simulink model "ReplayFlight_ALL_PARMS_v6"  (Simulink 7.5)
settings: Solver=FixedStepDiscrete  StartTime=0.0  StopTime=d_data(end,1)  FixedStep=apSampleTime  RelTol=1e-3
InitFcn:
  | replayFlight
values from neighbouring files (symbols this model uses):
  apSampleTime = 0.01    [demoz2SlugsV5.m]
  D = y    [BarOrthog.m]
  QUAT_0 = DCM2Quat( R0 )    [demoz2SlugsV5.m]
  R0 = single(Euler2DCMdeg( PHI_IC, THETA_IC, PSI_IC ))    [demoz2SlugsV5.m]
  SampleT = 0.02    [demoz2SlugsV5.m]
undefined symbols (not defined in the file or in its folder): aAxis_IC, accBiasRateLimit, accelXCutTemp, aPhi_IC, axTGain1, axTGain2, axTMean1, axTMean2, barAdjust, baroCutoff, baroCutTemp, baroOffset, baroScale, barTGain1, barTGain2, barTMean1, barTMean2, baseHeight, baseTemp, cubeAccelGain, cubeGyroGain, DiscIntNeverNeededParam, ePhi_IC, gaind, GS_location, gyroBiasRateLimit, Init_onlyOnce, Init_Reset, ISA_rho0, lapseRate, lowRateSensorCutoff, magMeanTemp, magOffset, magScale, magTempK, mainSensorCutoff, maxDynPressure, param_acc, param_mag, pitAdjust, pitCutTemp, pitotOffset, pitotScale, pitTGain1, pitTGain2, pitTMean1, pitTMean2, polesd, powerOffset, powerScale, pressureSensorCutoff, Psi_IC, T, tempOffset, tempScale, Theta_IC, Vb_0, vzCutoff, xCutoff, yCutoff ... (+2)
libraries: simulink x38, aerolibconvert2 x8, SLUGS_Library x6, dspmtrx3 x5, aerolibutil x4, dsPICdrivers x1
(part 4 of 5)

== system ReplayFlight_ALL_PARMS_v6/Position and Attitude Filter/Attitude Complimentary Filter COG/DoParmTests/DCM Tests/Create_OmegaBar ==
  w_curr : Inport
  w_prev : Inport  Port=2
  w_prev2 : Inport  Port=3
  2xapSampleTime : Constant  Value=2*apSampleTime  OutDataTypeMode=single  OutDataType=fixdt(1, 16)  OutScaling=2^0  OutDataTypeStr=single
  Const_2 : Constant  Value=2  OutDataTypeMode=single  OutDataType=fixdt(1, 16)  OutScaling=2^0  OutDataTypeStr=single
  Constant_1_2 : Constant  Value=1/2  OutDataTypeMode=single  OutDataType=fixdt(1, 16)  OutScaling=2^0  OutDataTypeStr=single
  Constant_1_6 : Constant  Value=1/6  OutDataTypeMode=single  OutDataType=fixdt(1, 16)  OutScaling=2^0  OutDataTypeStr=single
  Oddot : Product  Inputs=*/  OutDataType=fixdt(1, 16)  OutScaling=2^-10
  Odot : Product  Inputs=*/  OutDataType=fixdt(1, 16)  OutScaling=2^-10
  Product : Product  OutDataType=fixdt(1, 16)  OutScaling=2^0  RndMeth=Zero
  Product1 : Product  Inputs=3  OutDataType=fixdt(1, 16)  OutScaling=2^0  RndMeth=Zero
  Product2 : Product  Inputs=3  OutDataType=fixdt(1, 16)  OutScaling=2^0  RndMeth=Zero
  Product3 : Product  OutDataTypeMode=single  OutDataType=fixdt(1, 16)  OutScaling=2^0  OutDataTypeStr=single  SampleTime=apSampleTime  RndMeth=Zero
  SampleTime_sqrd : Constant  Value=apSampleTime^2  OutDataTypeMode=single  OutDataType=fixdt(1, 16)  OutScaling=2^0  OutDataTypeStr=single
  Subtract : Sum  Inputs=+-  OutDataType=fixdt(1, 16)  OutScaling=2^-10
  Subtract1 : Sum  Inputs=+-+  OutDataType=fixdt(1, 16)  OutScaling=2^-10
  Subtract2 : Sum  Inputs=+++  OutDataTypeMode=single  OutDataType=fixdt(1, 16)  OutScaling=2^-10  OutDataTypeStr=single
  apSampleTime : Constant  Value=apSampleTime  OutDataTypeMode=single  OutDataType=fixdt(1, 16)  OutScaling=2^0  OutDataTypeStr=single
  OmegaBar : Outport
  wires:
  Product2/1 -> Subtract2/3
  Oddot/1 -> Product2/2
  Product3/1 -> Product2/1
  Constant_1_6/1 -> Product2/3
  Product1/1 -> Subtract2/2
  Odot/1 -> Product1/3
  apSampleTime/1 -> Product3/2, Product3/1, Product1/2
  Constant_1_2/1 -> Product1/1
  Subtract2/1 -> OmegaBar/1
  Product/1 -> Subtract1/2
  Const_2/1 -> Product/2
  Subtract1/1 -> Oddot/1
  SampleTime_sqrd/1 -> Oddot/2
  2xapSampleTime/1 -> Odot/2
  Subtract/1 -> Odot/1
  w_prev2/1 -> Subtract1/3, Subtract/2
  w_curr/1 -> Subtract1/1, Subtract/1
  w_prev/1 -> Subtract2/1, Product/1

== system ReplayFlight_ALL_PARMS_v6/Position and Attitude Filter/Attitude Complimentary Filter COG/DoParmTests/DCM Tests/Murray_Mexp ==
  w_in : Inport  OutDataType=fixdt(1, 16)  OutScaling=2^0
  R_prev : Inport  Port=2  OutDataType=fixdt(1, 16)  OutScaling=2^0
  Add : Sum  Inputs=+++  OutDataTypeMode=single  OutDataType=fixdt(1, 16)  OutScaling=2^-10  OutDataTypeStr=single  SampleTime=apSampleTime
  Cosine_X : Trigonometry  Operator=cos
  Divide : Product  Inputs=*/  OutDataType=fixdt(1, 16)  OutScaling=2^-10
  Divide1 : Product  Inputs=*/  OutDataType=fixdt(1, 16)  OutScaling=2^-10
  Embedded MATLAB Function : Stateflow chart  TreatAsAtomicUnit=on
  Identity Matrix : dspmtrx3/Identity Matrix  Inherit=off  N=3  Ts=apSampleTime  dataType=single  isSigned=on  wordLen=16  udDataType=sfix(16)  fracBitsMode=Best precision  numFracBits=15
  Identity Matrix1 : dspmtrx3/Identity Matrix  Inherit=off  N=3  Ts=apSampleTime  dataType=single  isSigned=on  wordLen=16  udDataType=sfix(16)  fracBitsMode=Best precision  numFracBits=15
  Matrix Multiply1 : Product  Multiplication=Matrix(*)  OutDataType=sfix(16)  OutScaling=2^0
  Matrix Multiply2 : Product  Multiplication=Matrix(*)  OutDataType=sfix(16)  OutScaling=2^0
  Product{,1..3} (4 alike) : Product  OutDataType=fixdt(1, 16)  OutScaling=2^0  RndMeth=Zero
  Rexp : Switch  Criteria=u2 ~= 0  OutDataType=fixdt(1, 16)  OutScaling=2^0
  Sine_X : Trigonometry
  Skew symmetric matrix : Subsystem
  Subtract : Sum  Inputs=+-  OutDataType=fixdt(1, 16)  OutScaling=2^-10
  apSampleTime : Constant  Value=apSampleTime  OutDataTypeMode=single  OutDataType=fixdt(1, 16)  OutScaling=2^0  OutDataTypeStr=single
  apSampleTime1 : Constant  OutDataTypeMode=single  OutDataType=fixdt(1, 16)  OutScaling=2^0  OutDataTypeStr=single
  DCM_out : Outport  OutDataType=fixdt(1, 16)  OutScaling=2^0
  wires:
  Rexp/1 -> Matrix Multiply1/2
  Identity Matrix1/1 -> Rexp/3
  Add/1 -> Rexp/1
  Matrix Multiply1/1 -> DCM_out/1
  R_prev/1 -> Matrix Multiply1/1
  Product3/1 -> Add/2
  Divide/1 -> Product3/2
  Sine_X/1 -> Divide/1
  Product2/1 -> Add/3
  Matrix Multiply2/1 -> Product2/1
  Divide1/1 -> Product2/2
  Product1/1 -> Divide1/2
  Subtract/1 -> Divide1/1
  Cosine_X/1 -> Subtract/2
  apSampleTime1/1 -> Subtract/1
  Skew symmetric matrix/1(omega_x) -> Product3/1, Matrix Multiply2/2, Matrix Multiply2/1
  Product/1 -> Sine_X/1, Cosine_X/1
  apSampleTime/1 -> Product/2
  Embedded MATLAB Function/1(y) -> Rexp/2, Divide/2, Product1/1, Product1/2, Product/1
  Identity Matrix/1 -> Add/1
  w_in/1 -> Embedded MATLAB Function/1(u), Skew symmetric matrix/1(omega_in)

== system ReplayFlight_ALL_PARMS_v6/Position and Attitude Filter/Attitude Complimentary Filter COG/DoParmTests/DCM Tests/Skew symmetric matrix ==
  omega_in : Inport  PortDimensions=3  SampleTime=SampleT  OutDataType=fixdt(1, 16)  OutScaling=2^0
  Constant : Constant  Value=0  OutDataTypeMode=single  OutDataType=fixdt(1, 16)  OutScaling=2^0  OutDataTypeStr=single
  Constant1 : Constant  Value=0  OutDataTypeMode=single  OutDataType=fixdt(1, 16)  OutScaling=2^0  OutDataTypeStr=single
  Constant2 : Constant  Value=0  OutDataTypeMode=single  OutDataType=fixdt(1, 16)  OutScaling=2^0  OutDataTypeStr=single
  Demux : Demux  Outputs=3
  Gain : Gain  Gain=-1  ParameterDataType=fixdt(1, 16)  ParameterScaling=2^0  OutDataType=fixdt(1, 16)  OutScaling=2^0
  Gain1 : Gain  Gain=-1  ParameterDataType=fixdt(1, 16)  ParameterScaling=2^0  OutDataType=fixdt(1, 16)  OutScaling=2^0
  Gain2 : Gain  Gain=-1  ParameterDataType=fixdt(1, 16)  ParameterScaling=2^0  OutDataType=fixdt(1, 16)  OutScaling=2^0
  Mux{,1..3} (4 alike) : Mux  Inputs=3
  Reshape : Reshape  OutputDimensionality=Customize  OutputDimensions=[3,3]
  omega_x : Outport  PortDimensions=[3,3]  SampleTime=SampleT  OutDataType=fixdt(1, 16)  OutScaling=2^0
  wires:
  Gain2/1 -> Mux2/2
  Gain1/1 -> Mux1/1
  Gain/1 -> Mux/3
  Mux3/1 -> Reshape/1
  Mux2/1 -> Mux3/3
  Mux1/1 -> Mux3/2
  Mux/1 -> Mux3/1
  Constant2/1 -> Mux2/3
  Demux/1 -> Gain2/1, Mux1/3
  Constant1/1 -> Mux1/2
  Demux/2 -> Mux2/1, Gain/1
  Demux/3 -> Gain1/1, Mux/2
  Constant/1 -> Mux/1
  Reshape/1 -> omega_x/1
  omega_in/1 -> Demux/1

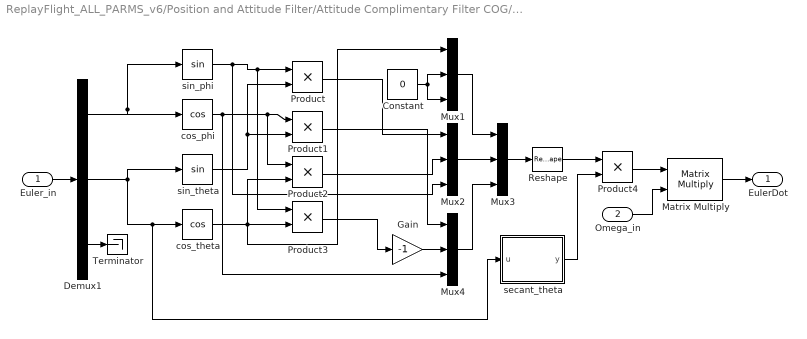
== system ReplayFlight_ALL_PARMS_v6/Position and Attitude Filter/Attitude Complimentary Filter COG/DoParmTests/Euler_Test/CreateEulerDot ==
  Euler_in : Inport  PortDimensions=3  SampleTime=SampleT  DataType=single  OutDataType=fixdt(1, 16)  OutScaling=2^0  OutDataTypeStr=single
  Omega_in : Inport  Port=2  PortDimensions=[3,1]  SampleTime=SampleT  DataType=single  OutDataType=fixdt(1, 16)  OutScaling=2^0  OutDataTypeStr=single
  Constant : Constant  Value=0  OutDataTypeMode=single  OutDataType=fixdt(1, 16)  OutScaling=2^0  OutDataTypeStr=single  SampleTime=SampleT
  Demux1 : Demux  Outputs=3
  Gain : Gain  Gain=-1  ParameterDataType=fixdt(1, 16)  ParameterScaling=2^0  OutDataTypeMode=single  OutDataType=fixdt(1, 16)  OutScaling=2^0  OutDataTypeStr=single  SampleTime=SampleT
  Matrix Multiply : Product  Multiplication=Matrix(*)  OutDataTypeMode=single  OutDataType=sfix(16)  OutScaling=2^0  OutDataTypeStr=single
  Mux{1..4} (4 alike) : Mux  Inputs=3
  Product{,1..3} (4 alike) : Product  OutDataTypeMode=single  OutDataType=fixdt(1, 16)  OutScaling=2^0  OutDataTypeStr=single  RndMeth=Zero
  Product4 : Product  OutDataTypeMode=single  OutDataType=fixdt(1, 16)  OutScaling=2^0  OutDataTypeStr=single  SampleTime=SampleT  RndMeth=Zero
  Reshape : Reshape  OutputDimensionality=Customize  OutputDimensions=[3,3]
  Terminator : Terminator
  cos_phi : Trigonometry  Operator=cos  SampleTime=SampleT
  cos_theta : Trigonometry  Operator=cos  SampleTime=SampleT
  secant_theta : Stateflow chart  TreatAsAtomicUnit=on
  sin_phi : Trigonometry  SampleTime=SampleT
  sin_theta : Trigonometry  SampleTime=SampleT
  EulerDot : Outport  DataType=single  OutDataType=fixdt(1, 16)  OutScaling=2^0  OutDataTypeStr=single
  wires:
  Product4/1 -> Matrix Multiply/1
  Reshape/1 -> Product4/1
  secant_theta/1(y) -> Product4/2
  Product3/1 -> Gain/1
  Gain/1 -> Mux4/2
  Product1/1 -> Mux4/1
  Product2/1 -> Mux2/2
  Product/1 -> Mux2/1
  Constant/1 -> Mux1/3, Mux1/2
  Mux4/1 -> Mux3/3
  Mux2/1 -> Mux3/2
  Mux1/1 -> Mux3/1
  Mux3/1 -> Reshape/1
  Omega_in/1 -> Matrix Multiply/2
  Matrix Multiply/1 -> EulerDot/1
  cos_theta/1 -> Mux1/1, Product3/2, Product2/2
  cos_phi/1 -> Mux4/3, Product2/1, Product1/1
  sin_theta/1 -> Product1/2, Product/2
  sin_phi/1 -> Mux2/3, Product3/1, Product/1
  Demux1/2 -> secant_theta/1(u), cos_theta/1, sin_theta/1
  Demux1/1 -> cos_phi/1, sin_phi/1
  Demux1/3 -> Terminator/1
  Euler_in/1 -> Demux1/1

== system ReplayFlight_ALL_PARMS_v6/Position and Attitude Filter/Attitude Complimentary Filter COG/DoParmTests/Euler_Test/Create_OmegaAverage ==
  In1 : Inport
  In2 : Inport  Port=2
  Add : Sum  OutDataType=fixdt(1, 16)  OutScaling=2^-10
  Constant : Constant  Value=2  OutDataTypeMode=single  OutDataType=fixdt(1, 16)  OutScaling=2^0  OutDataTypeStr=single
  Divide : Product  Inputs=*/  OutDataType=fixdt(1, 16)  OutScaling=2^-10
  Out1 : Outport
  wires:
  Constant/1 -> Divide/2
  Add/1 -> Divide/1
  In1/1 -> Add/1
  In2/1 -> Add/2
  Divide/1 -> Out1/1

== system ReplayFlight_ALL_PARMS_v6/Position and Attitude Filter/Attitude Complimentary Filter COG/DoParmTests/Euler_Test/Euler2DCM ==
  Euler_in : Inport  PortDimensions=3
  Create 3x3 Matrix : aerolibutil/Create 3x3 Matrix  SystemSampleTime=-1
  Fcn : Fcn  Expr=u(6)*u(5)  SampleTime=apSampleTime
  Fcn1 : Fcn  Expr=u(6)*u(2)*u(1)-u(3)*u(4)  SampleTime=apSampleTime
  Fcn2 : Fcn  Expr=u(6)*u(2)*u(4)+u(3)*u(1)  SampleTime=apSampleTime
  Fcn3 : Fcn  Expr=u(3)*u(5)  SampleTime=apSampleTime
  Fcn4 : Fcn  Expr=u(3)*u(2)*u(1)+u(6)*u(4)  SampleTime=apSampleTime
  Fcn5 : Fcn  Expr=u(3)*u(2)*u(4)-u(6)*u(1)  SampleTime=apSampleTime
  Fcn6 : Fcn  Expr=-u(2)  SampleTime=apSampleTime
  Fcn7 : Fcn  Expr=u(5)*u(1)  SampleTime=apSampleTime
  Fcn8 : Fcn  Expr=u(5)*u(4)  SampleTime=apSampleTime
  Mux1 : Mux  Inputs=2
  sincos : Trigonometry  Operator=sincos
  eDCM_out : Outport  PortDimensions=[3,3]
  wires:
  Euler_in/1 -> sincos/1
  sincos/1 -> Mux1/1
  sincos/2 -> Mux1/2
  Create 3x3 Matrix/1 -> eDCM_out/1
  Mux1/1 -> Fcn/1, Fcn1/1, Fcn2/1, Fcn3/1, Fcn4/1, Fcn5/1, Fcn8/1, Fcn7/1, Fcn6/1
  Fcn/1 -> Create 3x3 Matrix/1
  Fcn1/1 -> Create 3x3 Matrix/2
  Fcn2/1 -> Create 3x3 Matrix/3
  Fcn3/1 -> Create 3x3 Matrix/4
  Fcn4/1 -> Create 3x3 Matrix/5
  Fcn5/1 -> Create 3x3 Matrix/6
  Fcn6/1 -> Create 3x3 Matrix/7
  Fcn7/1 -> Create 3x3 Matrix/8
  Fcn8/1 -> Create 3x3 Matrix/9

== system ReplayFlight_ALL_PARMS_v6/Position and Attitude Filter/Attitude Complimentary Filter COG/DoParmTests/Quat_Test/Create_OmegaAverage ==
  In1 : Inport
  In2 : Inport  Port=2
  Add : Sum  OutDataType=fixdt(1, 16)  OutScaling=2^-10
  Constant : Constant  Value=2  OutDataTypeMode=single  OutDataType=fixdt(1, 16)  OutScaling=2^0  OutDataTypeStr=single
  Divide : Product  Inputs=*/  OutDataType=fixdt(1, 16)  OutScaling=2^-10
  Out1 : Outport
  wires:
  Constant/1 -> Divide/2
  Add/1 -> Divide/1
  In1/1 -> Add/1
  In2/1 -> Add/2
  Divide/1 -> Out1/1

== system ReplayFlight_ALL_PARMS_v6/Position and Attitude Filter/Attitude Complimentary Filter COG/DoParmTests/Quat_Test/Create_OmegaAverage1 ==
  In1 : Inport
  In2 : Inport  Port=2
  Add : Sum  OutDataType=fixdt(1, 16)  OutScaling=2^-10
  Constant : Constant  Value=2  OutDataTypeMode=single  OutDataType=fixdt(1, 16)  OutScaling=2^0  OutDataTypeStr=single
  Divide : Product  Inputs=*/  OutDataType=fixdt(1, 16)  OutScaling=2^-10
  Out1 : Outport
  wires:
  Divide/1 -> Out1/1
  In2/1 -> Add/2
  In1/1 -> Add/1
  Add/1 -> Divide/1
  Constant/1 -> Divide/2

== system ReplayFlight_ALL_PARMS_v6/Position and Attitude Filter/Attitude Complimentary Filter COG/DoParmTests/Quat_Test/Create_OmegaBar ==
  w_curr : Inport
  w_prev : Inport  Port=2
  w_prev2 : Inport  Port=3
  2xapSampleTime : Constant  Value=2*apSampleTime  OutDataTypeMode=single  OutDataType=fixdt(1, 16)  OutScaling=2^0  OutDataTypeStr=single
  Const_2 : Constant  Value=2  OutDataTypeMode=single  OutDataType=fixdt(1, 16)  OutScaling=2^0  OutDataTypeStr=single
  Constant_1_2 : Constant  Value=1/2  OutDataTypeMode=single  OutDataType=fixdt(1, 16)  OutScaling=2^0  OutDataTypeStr=single
  Constant_1_6 : Constant  Value=1/6  OutDataTypeMode=single  OutDataType=fixdt(1, 16)  OutScaling=2^0  OutDataTypeStr=single
  Oddot : Product  Inputs=*/  OutDataType=fixdt(1, 16)  OutScaling=2^-10
  Odot : Product  Inputs=*/  OutDataType=fixdt(1, 16)  OutScaling=2^-10
  Product : Product  OutDataType=fixdt(1, 16)  OutScaling=2^0  RndMeth=Zero
  Product1 : Product  Inputs=3  OutDataType=fixdt(1, 16)  OutScaling=2^0  RndMeth=Zero
  Product2 : Product  Inputs=3  OutDataType=fixdt(1, 16)  OutScaling=2^0  RndMeth=Zero
  Product3 : Product  OutDataTypeMode=single  OutDataType=fixdt(1, 16)  OutScaling=2^0  OutDataTypeStr=single  SampleTime=apSampleTime  RndMeth=Zero
  SampleTime_sqrd : Constant  Value=apSampleTime^2  OutDataTypeMode=single  OutDataType=fixdt(1, 16)  OutScaling=2^0  OutDataTypeStr=single
  Subtract : Sum  Inputs=+-  OutDataType=fixdt(1, 16)  OutScaling=2^-10
  Subtract1 : Sum  Inputs=+-+  OutDataType=fixdt(1, 16)  OutScaling=2^-10
  Subtract2 : Sum  Inputs=+++  OutDataTypeMode=single  OutDataType=fixdt(1, 16)  OutScaling=2^-10  OutDataTypeStr=single
  apSampleTime : Constant  Value=apSampleTime  OutDataTypeMode=single  OutDataType=fixdt(1, 16)  OutScaling=2^0  OutDataTypeStr=single
  OmegaBar : Outport
  wires:
  w_prev/1 -> Product/1, Subtract2/1
  w_curr/1 -> Subtract/1, Subtract1/1
  w_prev2/1 -> Subtract/2, Subtract1/3
  Subtract/1 -> Odot/1
  2xapSampleTime/1 -> Odot/2
  SampleTime_sqrd/1 -> Oddot/2
  Subtract1/1 -> Oddot/1
  Const_2/1 -> Product/2
  Product/1 -> Subtract1/2
  Subtract2/1 -> OmegaBar/1
  Constant_1_2/1 -> Product1/1
  apSampleTime/1 -> Product1/2, Product3/1, Product3/2
  Odot/1 -> Product1/3
  Product1/1 -> Subtract2/2
  Constant_1_6/1 -> Product2/3
  Product3/1 -> Product2/1
  Oddot/1 -> Product2/2
  Product2/1 -> Subtract2/3

== system ReplayFlight_ALL_PARMS_v6/Position and Attitude Filter/Attitude Complimentary Filter COG/DoParmTests/Quat_Test/Quat_Mexp_Wertz ==
  note: Model implements quaternion-based matrix exponential propagation of attitude.
      | Omega = [ 0 -p -q -r; p 0 r -q; q -r 0 p; r q -p 0 ];
      | wn = sqrt( p^2 + q^2 + r^2 );
      |
      | % Closed-form integration
      | if( wn ~= 0 )
      |     Q_next = (   cos( wn * dt / 2 ) * I4 + ...
      |         (1/wn) * sin( wn * dt / 2 ) * Omega ) * q_in;
      | else
      |     Q_next = q_in; % (wn == 0) --> no change in q_in
      | end
  w_in : Inport  OutDataType=fixdt(1, 16)  OutScaling=2^0
  q_in : Inport  Port=2  OutDataType=fixdt(1, 16)  OutScaling=2^0
  1_by_wn : Product  Inputs=*/  OutDataType=fixdt(1, 16)  OutScaling=2^-10
  Add : Sum  OutDataTypeMode=single  OutDataType=fixdt(1, 16)  OutScaling=2^-10  OutDataTypeStr=single  SampleTime=apSampleTime
  Constant1 : Constant  OutDataTypeMode=single  OutDataType=fixdt(1, 16)  OutScaling=2^0  OutDataTypeStr=single
  Constant2 : Constant  Value=2  OutDataTypeMode=single  OutDataType=fixdt(1, 16)  OutScaling=2^0  OutDataTypeStr=single
  Cosine_X : Trigonometry  Operator=cos
  Embedded MATLAB Function : Stateflow chart  TreatAsAtomicUnit=on
  Identity Matrix : dspmtrx3/Identity Matrix  Inherit=off  N=4  Ts=apSampleTime  dataType=single  isSigned=on  wordLen=16  udDataType=sfix(16)  fracBitsMode=Best precision  numFracBits=15
  Qexp : Product  Multiplication=Matrix(*)  OutDataTypeMode=single  OutDataType=sfix(16)  OutScaling=2^0  OutDataTypeStr=single  SampleTime=SampleT
  Sine_X : Trigonometry
  Skew symmetric matrix1 : Subsystem
  Switch_on_wn : Switch  Criteria=u2 ~= 0  OutDataTypeMode=single  OutDataType=fixdt(1, 16)  OutScaling=2^0  OutDataTypeStr=single
  apSampleTime : Constant  Value=apSampleTime  OutDataTypeMode=single  OutDataType=fixdt(1, 16)  OutScaling=2^0  OutDataTypeStr=single
  wn_dt{,1..3} (4 alike) : Product  OutDataType=fixdt(1, 16)  OutScaling=2^0  RndMeth=Zero
  wn_dt_by_2 : Product  Inputs=*/  OutDataType=fixdt(1, 16)  OutScaling=2^-10
  q_out : Outport  OutDataType=fixdt(1, 16)  OutScaling=2^0
  wires:
  Embedded MATLAB Function/1(y) -> wn_dt/1, 1_by_wn/2, Switch_on_wn/2
  apSampleTime/1 -> wn_dt/2
  w_in/1 -> Embedded MATLAB Function/1(u), Skew symmetric matrix1/1(omega_in)
  wn_dt/1 -> wn_dt_by_2/1
  Constant2/1 -> wn_dt_by_2/2
  wn_dt_by_2/1 -> Sine_X/1, Cosine_X/1
  Constant1/1 -> 1_by_wn/1
  Sine_X/1 -> wn_dt1/2
  1_by_wn/1 -> wn_dt1/1
  wn_dt1/1 -> wn_dt3/2
  wn_dt3/1 -> Add/1
  Cosine_X/1 -> wn_dt2/1
  Identity Matrix/1 -> wn_dt2/2
  wn_dt2/1 -> Add/2
  Skew symmetric matrix1/1(omega_x) -> wn_dt3/1
  Qexp/1 -> Switch_on_wn/1
  Add/1 -> Qexp/1
  q_in/1 -> Qexp/2, Switch_on_wn/3
  Switch_on_wn/1 -> q_out/1

== system ReplayFlight_ALL_PARMS_v6/Position and Attitude Filter/Attitude Complimentary Filter COG/DoParmTests/Quat_Test/Quaternions to  Direction Cosine Matrix ==
  Quat : Inport  PortDimensions=4  OutDataType=sfix(16)  OutScaling=2^0
  A11 : Subsystem
  A12 : Subsystem
  A13 : Subsystem
  A21 : Subsystem
  A22 : Subsystem
  A23 : Subsystem
  A31 : Subsystem
  A32 : Subsystem
  A33 : Subsystem
  Create Transformation Matrix : Subsystem  AncestorBlock=aerolibutil/Create 3x3 Matrix  mask(Create 3x3 Matrix){}
      mask help:
      | Create a 3-by-3 matrix from nine input values. Each input corresponds to an element of the matrix.
      |
      | For example, the input labeled A21 is the entry in the second row and first column of the matrix.
      mask init:
      | aeroicon('aeroblk');
      mask Help: web(asbhelp);
      mask Display:
      | port_label('input',1,'A_{11}','texmode','on');
      | port_label('input',2,'A_{12}','texmode','on');
      | port_label('input',3,'A_{13}','texmode','on');
      | port_label('input',4,'A_{21}','texmode','on');
      | port_label('input',5,'A_{22}','texmode','on');
      | port_label('input',6,'A_{23}','texmode','on');
      | port_label('input',7,'A_{31}','texmode','on');
      | port_label('input',8,'A_{32}','texmode','on');
      | port_label('input',9,'A_{33}','texmode','on');
      | port_label('output',1,'A','texmode','on');
  DCM : Outport  PortDimensions=[3,3]  OutDataType=sfix(16)  OutScaling=2^0  InitialOutput=0
  wires:
  Create Transformation Matrix/1(Matrix) -> DCM/1
  A11/1(A11) -> Create Transformation Matrix/1(M11)
  A21/1(A21) -> Create Transformation Matrix/4(M21)
  A31/1(A31) -> Create Transformation Matrix/7(M31)
  A32/1(A32) -> Create Transformation Matrix/8(M32)
  A13/1(A13) -> Create Transformation Matrix/3(M13)
  A23/1(A23) -> Create Transformation Matrix/6(M23)
  A33/1(A33) -> Create Transformation Matrix/9(M33)
  Quat/1 -> A33/1(normal(q)), A32/1(normal(q)), A31/1(normal(q)), A23/1(normal(q)), A22/1(normal(q)), A21/1(normal(q)), A13/1(normal(q)), A12/1(normal(q)), A11/1(normal(q))
  A22/1(A22) -> Create Transformation Matrix/5(M22)
  A12/1(A12) -> Create Transformation Matrix/2(M12)

== system ReplayFlight_ALL_PARMS_v6/Position and Attitude Filter/Attitude Complimentary Filter COG/DoParmTests/Quat_Test/Skew symmetric matrix ==
  omega_in : Inport  DataType=single  OutDataType=fixdt(1, 16)  OutScaling=2^0  OutDataTypeStr=single
  Constant{1..4} (4 alike) : Constant  Value=0  OutDataTypeMode=single  OutDataType=fixdt(1, 16)  OutScaling=2^0  OutDataTypeStr=single
  Demux : Demux  Outputs=3
  Gain1 : Gain  Gain=-1  ParameterDataType=fixdt(1, 16)  ParameterScaling=2^0  OutDataTypeMode=single  OutDataType=fixdt(1, 16)  OutScaling=2^0  OutDataTypeStr=single
  Gain2 : Gain  Gain=-1  ParameterDataType=fixdt(1, 16)  ParameterScaling=2^0  OutDataTypeMode=single  OutDataType=fixdt(1, 16)  OutScaling=2^0  OutDataTypeStr=single
  Gain3 : Gain  Gain=-1  ParameterDataType=fixdt(1, 16)  ParameterScaling=2^0  OutDataTypeMode=single  OutDataType=fixdt(1, 16)  OutScaling=2^0  OutDataTypeStr=single
  Mux{,1..4} (5 alike) : Mux
  Reshape : Reshape  OutputDimensionality=Customize  OutputDimensions=[4,4]
  omega_x : Outport  DataType=single  OutDataType=fixdt(1, 16)  OutScaling=2^0  OutDataTypeStr=single
  wires:
  Gain1/1 -> Mux4/2, Mux2/1
  Gain3/1 -> Mux4/1, Mux1/3
  Gain2/1 -> Mux2/4, Mux1/1
  Mux3/1 -> Reshape/1
  Reshape/1 -> omega_x/1
  omega_in/1 -> Demux/1
  Mux/1 -> Mux3/1
  Mux1/1 -> Mux3/2
  Mux2/1 -> Mux3/3
  Mux4/1 -> Mux3/4
  Constant4/1 -> Mux4/4
  Constant2/1 -> Mux2/3
  Constant1/1 -> Mux1/2
  Constant3/1 -> Mux/1
  Demux/1 -> Mux4/3, Mux/2, Gain2/1
  Demux/2 -> Mux1/4, Mux/3, Gain1/1
  Demux/3 -> Mux2/2, Mux/4, Gain3/1

== system ReplayFlight_ALL_PARMS_v6/Position and Attitude Filter/Geod2LTP1/ECEF2LTP (UEN)/From Body to Universal1/Rotation Matrix from Long//Lat ==
  note: Calculate Coefficients of DCM Row-Wise
  long lat : Inport  OutDataType=sfix(16)  OutScaling=2^0
  11 : Fcn  Expr=cos(u[1])*cos(u[2])
  12 : Fcn  Expr=sin(u[1])*cos(u[2])
  13 : Fcn  Expr=sin(u[2])
  21 : Fcn  Expr=-sin(u[1])
  22 : Fcn  Expr=cos(u[1])
  23 : Fcn  Expr=0
  31 : Fcn  Expr=-sin(u[2])*cos(u[1])
  32 : Fcn  Expr=-sin(u[1])*sin(u[2])
  33 : Fcn  Expr=cos(u[2])
  Mux2 : Mux  Inputs=9
  DCM : Outport  OutDataType=sfix(16)  OutScaling=2^0  InitialOutput=0
  wires:
  33/1 -> Mux2/9
  23/1 -> Mux2/8
  13/1 -> Mux2/7
  32/1 -> Mux2/6
  22/1 -> Mux2/5
  12/1 -> Mux2/4
  31/1 -> Mux2/3
  21/1 -> Mux2/2
  11/1 -> Mux2/1
  Mux2/1 -> DCM/1
  long lat/1 -> 11/1, 33/1, 23/1, 13/1, 32/1, 22/1, 12/1, 31/1, 21/1

== system ReplayFlight_ALL_PARMS_v6/Position and Attitude Filter/Position Filter/BlendPosVel/1D Filter/Filter2 ==
  In1 : Inport  OutDataType=sfix(16)  OutScaling=2^0
  Discrete Zero-Pole : DiscreteZeroPole  Zeros=zerosd  Poles=polesd  Gain=gaind  SampleTime=SampleTime
  Out1 : Outport  OutDataType=sfix(16)  OutScaling=2^0
  wires:
  Discrete Zero-Pole/1 -> Out1/1
  In1/1 -> Discrete Zero-Pole/1

== system ReplayFlight_ALL_PARMS_v6/Position and Attitude Filter/Position Filter/BlendPosVel/1D Filter2/Filter2 ==
  In1 : Inport  OutDataType=sfix(16)  OutScaling=2^0
  Discrete Zero-Pole : DiscreteZeroPole  Zeros=zerosd  Poles=polesd  Gain=gaind  SampleTime=SampleTime
  Out1 : Outport  OutDataType=sfix(16)  OutScaling=2^0
  wires:
  Discrete Zero-Pole/1 -> Out1/1
  In1/1 -> Discrete Zero-Pole/1

== system ReplayFlight_ALL_PARMS_v6/Position and Attitude Filter/Position Filter/BlendPosVel/2 FIlter Blend/1D Filter ==
  In1 : Inport  OutDataType=sfix(16)  OutScaling=2^0
  Data Type Conversion1 : DataTypeConversion  OutDataTypeMode=single  OutDataType=sfix(16)  OutScaling=2^0  OutDataTypeStr=single
  Data Type Conversion2 : DataTypeConversion  OutDataTypeMode=double  OutDataType=sfix(16)  OutScaling=2^0  OutDataTypeStr=double
  Filter2 : Subsystem  mask(DiscretizedZeroPole){Zeros=zval, Poles=pval, Gain=kval, AbsTol=auto, SampleTime=TSample, method=tustin, Wc=1}
      mask prompts: Zeros "Zeros (enter in s-main:)"; Poles "Poles (enter in s-domain:)"; Gain "Gain (enter in s-domain:)"; AbsTol "Absolute tolerance:"; SampleTime "Sample time:"; Wc "Critical Frequency (Hz):"
      mask help: Continuous mask uses c2d to transform parameters onto the Discrete Zero-Pole block inside.
      mask init: same as ReplayFlight_ALL_PARMS_v6/Position and Attitude Filter/Attitude Complimentary Filter COG/3D Filter/Filter1
      mask StyleString: edit,edit,edit,edit,edit,popup(zoh|foh|tustin|prewarp|matched),edit
      mask CallbackString: |||||hidecrit|
      mask Display:
      | droots(zeross,poless,gainss)
      | text( 0.5, 1.0, method, 'verticalAlignment','top')
  Out1 : Outport  OutDataType=sfix(16)  OutScaling=2^0
  wires:
  Data Type Conversion1/1 -> Out1/1
  Data Type Conversion2/1 -> Filter2/1(In1)
  In1/1 -> Data Type Conversion2/1
  Filter2/1(Out1) -> Data Type Conversion1/1

== system ReplayFlight_ALL_PARMS_v6/Position and Attitude Filter/Position Filter/BlendPosVel/2 FIlter Blend/1D Filter1 ==
  In1 : Inport  OutDataType=sfix(16)  OutScaling=2^0
  Data Type Conversion1 : DataTypeConversion  OutDataTypeMode=single  OutDataType=sfix(16)  OutScaling=2^0  OutDataTypeStr=single
  Data Type Conversion2 : DataTypeConversion  OutDataTypeMode=double  OutDataType=sfix(16)  OutScaling=2^0  OutDataTypeStr=double
  Filter2 : Subsystem  mask(DiscretizedZeroPole){Zeros=zval, Poles=pval, Gain=kval, AbsTol=auto, SampleTime=TSample, method=tustin, Wc=1}
      mask prompts: Zeros "Zeros (enter in s-main:)"; Poles "Poles (enter in s-domain:)"; Gain "Gain (enter in s-domain:)"; AbsTol "Absolute tolerance:"; SampleTime "Sample time:"; Wc "Critical Frequency (Hz):"
      mask help: Continuous mask uses c2d to transform parameters onto the Discrete Zero-Pole block inside.
      mask init: same as ReplayFlight_ALL_PARMS_v6/Position and Attitude Filter/Attitude Complimentary Filter COG/3D Filter/Filter1
      mask StyleString: edit,edit,edit,edit,edit,popup(zoh|foh|tustin|prewarp|matched),edit
      mask CallbackString: |||||hidecrit|
      mask Display:
      | droots(zeross,poless,gainss)
      | text( 0.5, 1.0, method, 'verticalAlignment','top')
  Out1 : Outport  OutDataType=sfix(16)  OutScaling=2^0
  wires:
  Filter2/1(Out1) -> Data Type Conversion1/1
  In1/1 -> Data Type Conversion2/1
  Data Type Conversion2/1 -> Filter2/1(In1)
  Data Type Conversion1/1 -> Out1/1

== system ReplayFlight_ALL_PARMS_v6/Position and Attitude Filter/Position Filter/BlendPosVel/3D Filter/Filter1 ==
  In1 : Inport  OutDataType=sfix(16)  OutScaling=2^0
  Discrete Zero-Pole : DiscreteZeroPole  Zeros=zerosd  Poles=polesd  Gain=gaind  SampleTime=SampleTime
  Out1 : Outport  OutDataType=sfix(16)  OutScaling=2^0
  wires:
  In1/1 -> Discrete Zero-Pole/1
  Discrete Zero-Pole/1 -> Out1/1

== system ReplayFlight_ALL_PARMS_v6/Position and Attitude Filter/Position Filter/BlendPosVel/3D Filter/Filter2 ==
  In1 : Inport  OutDataType=sfix(16)  OutScaling=2^0
  Discrete Zero-Pole : DiscreteZeroPole  Zeros=zerosd  Poles=polesd  Gain=gaind  SampleTime=SampleTime
  Out1 : Outport  OutDataType=sfix(16)  OutScaling=2^0
  wires:
  Discrete Zero-Pole/1 -> Out1/1
  In1/1 -> Discrete Zero-Pole/1

== system ReplayFlight_ALL_PARMS_v6/Position and Attitude Filter/Position Filter/BlendPosVel/3D Filter/Filter3 ==
  In1 : Inport  OutDataType=sfix(16)  OutScaling=2^0
  Discrete Zero-Pole : DiscreteZeroPole  Zeros=zerosd  Poles=polesd  Gain=gaind  SampleTime=SampleTime
  Out1 : Outport  OutDataType=sfix(16)  OutScaling=2^0
  wires:
  In1/1 -> Discrete Zero-Pole/1
  Discrete Zero-Pole/1 -> Out1/1

== system ReplayFlight_ALL_PARMS_v6/Position and Attitude Filter/Position Filter/BlendPosVel/CompFiltRate/1D Filter1 ==
  In1 : Inport  OutDataType=sfix(16)  OutScaling=2^0
  Data Type Conversion1 : DataTypeConversion  OutDataTypeMode=single  OutDataType=sfix(16)  OutScaling=2^0  OutDataTypeStr=single
  Data Type Conversion2 : DataTypeConversion  OutDataTypeMode=double  OutDataType=sfix(16)  OutScaling=2^0  OutDataTypeStr=double
  Filter2 : Subsystem  mask(DiscretizedZeroPole){Zeros=zval, Poles=pval, Gain=kval, AbsTol=auto, SampleTime=TSample, method=tustin, Wc=1}
      mask prompts: Zeros "Zeros (enter in s-main:)"; Poles "Poles (enter in s-domain:)"; Gain "Gain (enter in s-domain:)"; AbsTol "Absolute tolerance:"; SampleTime "Sample time:"; Wc "Critical Frequency (Hz):"
      mask help: Continuous mask uses c2d to transform parameters onto the Discrete Zero-Pole block inside.
      mask init: same as ReplayFlight_ALL_PARMS_v6/Position and Attitude Filter/Attitude Complimentary Filter COG/3D Filter/Filter1
      mask StyleString: edit,edit,edit,edit,edit,popup(zoh|foh|tustin|prewarp|matched),edit
      mask CallbackString: |||||hidecrit|
      mask Display:
      | droots(zeross,poless,gainss)
      | text( 0.5, 1.0, method, 'verticalAlignment','top')
  Out1 : Outport  OutDataType=sfix(16)  OutScaling=2^0
  wires:
  Filter2/1(Out1) -> Data Type Conversion1/1
  In1/1 -> Data Type Conversion2/1
  Data Type Conversion2/1 -> Filter2/1(In1)
  Data Type Conversion1/1 -> Out1/1

== system ReplayFlight_ALL_PARMS_v6/Position and Attitude Filter/Position Filter/BlendPosVel/CompFiltRate1/1D Filter1 ==
  In1 : Inport  OutDataType=sfix(16)  OutScaling=2^0
  Data Type Conversion1 : DataTypeConversion  OutDataTypeMode=single  OutDataType=sfix(16)  OutScaling=2^0  OutDataTypeStr=single
  Data Type Conversion2 : DataTypeConversion  OutDataTypeMode=double  OutDataType=sfix(16)  OutScaling=2^0  OutDataTypeStr=double
  Filter2 : Subsystem  mask(DiscretizedZeroPole){Zeros=zval, Poles=pval, Gain=kval, AbsTol=auto, SampleTime=TSample, method=tustin, Wc=1}
      mask prompts: Zeros "Zeros (enter in s-main:)"; Poles "Poles (enter in s-domain:)"; Gain "Gain (enter in s-domain:)"; AbsTol "Absolute tolerance:"; SampleTime "Sample time:"; Wc "Critical Frequency (Hz):"
      mask help: Continuous mask uses c2d to transform parameters onto the Discrete Zero-Pole block inside.
      mask init: same as ReplayFlight_ALL_PARMS_v6/Position and Attitude Filter/Attitude Complimentary Filter COG/3D Filter/Filter1
      mask StyleString: edit,edit,edit,edit,edit,popup(zoh|foh|tustin|prewarp|matched),edit
      mask CallbackString: |||||hidecrit|
      mask Display:
      | droots(zeross,poless,gainss)
      | text( 0.5, 1.0, method, 'verticalAlignment','top')
  Out1 : Outport  OutDataType=sfix(16)  OutScaling=2^0
  wires:
  Filter2/1(Out1) -> Data Type Conversion1/1
  In1/1 -> Data Type Conversion2/1
  Data Type Conversion2/1 -> Filter2/1(In1)
  Data Type Conversion1/1 -> Out1/1

== system ReplayFlight_ALL_PARMS_v6/Position and Attitude Filter/Position Filter/BlendPosVel/CompRateOnly/1D Filter1 ==
  In1 : Inport  OutDataType=sfix(16)  OutScaling=2^0
  Data Type Conversion1 : DataTypeConversion  OutDataTypeMode=single  OutDataType=sfix(16)  OutScaling=2^0  OutDataTypeStr=single
  Data Type Conversion2 : DataTypeConversion  OutDataTypeMode=double  OutDataType=sfix(16)  OutScaling=2^0  OutDataTypeStr=double
  Filter2 : Subsystem  mask(DiscretizedZeroPole){Zeros=zval, Poles=pval, Gain=kval, AbsTol=auto, SampleTime=TSample, method=tustin, Wc=1}
      mask prompts: Zeros "Zeros (enter in s-main:)"; Poles "Poles (enter in s-domain:)"; Gain "Gain (enter in s-domain:)"; AbsTol "Absolute tolerance:"; SampleTime "Sample time:"; Wc "Critical Frequency (Hz):"
      mask help: Continuous mask uses c2d to transform parameters onto the Discrete Zero-Pole block inside.
      mask init: same as ReplayFlight_ALL_PARMS_v6/Position and Attitude Filter/Attitude Complimentary Filter COG/3D Filter/Filter1
      mask StyleString: edit,edit,edit,edit,edit,popup(zoh|foh|tustin|prewarp|matched),edit
      mask CallbackString: |||||hidecrit|
      mask Display:
      | droots(zeross,poless,gainss)
      | text( 0.5, 1.0, method, 'verticalAlignment','top')
  Out1 : Outport  OutDataType=sfix(16)  OutScaling=2^0
  wires:
  Filter2/1(Out1) -> Data Type Conversion1/1
  In1/1 -> Data Type Conversion2/1
  Data Type Conversion2/1 -> Filter2/1(In1)
  Data Type Conversion1/1 -> Out1/1

== system ReplayFlight_ALL_PARMS_v6/Sensor Data/Sensor Suite/Cube Signal Cond/Temp Compensate Accel X/Hi Temp Compensation ==
  Raw : Inport  OutDataType=sfix(16)  OutScaling=2^0
  Temp Raw : Inport  Port=2  OutDataType=sfix(16)  OutScaling=2^0
  Enable : EnablePort
  Divide1 : Product  OutDataTypeMode=single  OutDataType=sfix(16)  OutScaling=2^-10  OutDataTypeStr=single
  Mean Temperature for Calibration : Constant  Value=tempMean  OutDataTypeMode=single  OutDataType=sfix(16)  OutScaling=2^0  OutDataTypeStr=single
  Sum1 : Sum  Inputs=|+-  OutDataTypeMode=single  OutDataType=sfix(16)  OutScaling=2^0  OutDataTypeStr=single
  Sum2 : Sum  Inputs=|+-  OutDataTypeMode=single  OutDataType=sfix(16)  OutScaling=2^0  OutDataTypeStr=single
  gains : Constant  Value=alpha  OutDataTypeMode=single  OutDataType=sfix(16)  OutScaling=2^0  OutDataTypeStr=single
  Comp : Outport  OutDataType=sfix(16)  OutScaling=2^0
  wires:
  Mean Temperature for Calibration/1 -> Sum1/2
  Raw/1 -> Sum2/1
  Temp Raw/1 -> Sum1/1
  Sum1/1 -> Divide1/2
  gains/1 -> Divide1/1
  Divide1/1 -> Sum2/2
  Sum2/1 -> Comp/1

== system ReplayFlight_ALL_PARMS_v6/Sensor Data/Sensor Suite/Cube Signal Cond/Temp Compensate Accel X/Lo Temp Compensation ==
  Raw : Inport  OutDataType=sfix(16)  OutScaling=2^0
  Temp Raw : Inport  Port=2  OutDataType=sfix(16)  OutScaling=2^0
  Enable : EnablePort
  Divide1 : Product  OutDataTypeMode=single  OutDataType=sfix(16)  OutScaling=2^-10  OutDataTypeStr=single
  Mean Temperature for Calibration : Constant  Value=tempMean  OutDataTypeMode=single  OutDataType=sfix(16)  OutScaling=2^0  OutDataTypeStr=single
  Sum1 : Sum  Inputs=|+-  OutDataTypeMode=single  OutDataType=sfix(16)  OutScaling=2^0  OutDataTypeStr=single
  Sum2 : Sum  Inputs=|+-  OutDataTypeMode=single  OutDataType=sfix(16)  OutScaling=2^0  OutDataTypeStr=single
  gains : Constant  Value=alpha  OutDataTypeMode=single  OutDataType=sfix(16)  OutScaling=2^0  OutDataTypeStr=single
  Comp : Outport  OutDataType=sfix(16)  OutScaling=2^0
  wires:
  Sum2/1 -> Comp/1
  Divide1/1 -> Sum2/2
  gains/1 -> Divide1/1
  Sum1/1 -> Divide1/2
  Temp Raw/1 -> Sum1/1
  Raw/1 -> Sum2/1
  Mean Temperature for Calibration/1 -> Sum1/2

== system ReplayFlight_ALL_PARMS_v6/Sensor Data/Sensor Suite/Low Pass Filtering,Temperature Compensation and Calibration/Baro Altimeter/Compute Barometric Height ==
  Base Height (m) : Inport  OutDataType=sfix(16)  OutScaling=2^0
  Base Pressure (Pa) : Inport  Port=2  OutDataType=sfix(16)  OutScaling=2^0
  Baro (Pa) : Inport  Port=3  OutDataType=sfix(16)  OutScaling=2^0
  Constant2 : Constant  Value=baseTemp/(-LapseRate)  OutDataTypeMode=single  OutDataType=sfix(16)  OutScaling=2^0  OutDataTypeStr=single
  Constant3 : Constant  Value=9.350253e-2  OutDataTypeMode=single  OutDataType=sfix(16)  OutScaling=2^0  OutDataTypeStr=single
  Constant4 : Constant  Value=-1.888933e-1  OutDataTypeMode=single  OutDataType=sfix(16)  OutScaling=2^0  OutDataTypeStr=single
  Constant5 : Constant  Value=2.180313e-5  OutDataTypeMode=single  OutDataType=sfix(16)  OutScaling=2^0  OutDataTypeStr=single
  Divide : Product  Inputs=*/  OutDataTypeMode=single  OutDataType=sfix(16)  OutScaling=2^-10  OutDataTypeStr=single
  Divide{1..4} (4 alike) : Product  OutDataTypeMode=single  OutDataType=sfix(16)  OutScaling=2^-10  OutDataTypeStr=single
  Length Conversion : aerolibconvert2/Length Conversion  SystemSampleTime=-1  IU=ft  OU=m
  Sum1 : Sum  Inputs=|++  OutDataTypeMode=single  OutDataType=sfix(16)  OutScaling=2^0  OutDataTypeStr=single
  Sum2 : Sum  Inputs=|+-  OutDataTypeMode=single  OutDataType=sfix(16)  OutScaling=2^0  OutDataTypeStr=single
  Sum3 : Sum  Inputs=3  OutDataTypeMode=single  OutDataType=sfix(16)  OutScaling=2^0  OutDataTypeStr=single
  "Altitude, m" : Outport  OutDataType=sfix(16)  OutScaling=2^0
  wires:
  Baro (Pa)/1 -> Sum2/1
  Base Height (m)/1 -> Sum1/2
  Base Pressure (Pa)/1 -> Sum2/2, Divide/2
  Divide/1 -> Divide4/2, Divide4/1, Divide2/1  "x"
  Divide4/1 -> Divide1/1  "x^2"
  Constant3/1 -> Divide1/2
  Constant4/1 -> Divide2/2
  Divide1/1 -> Sum3/1
  Divide2/1 -> Sum3/2
  Constant5/1 -> Sum3/3
  Sum3/1 -> Divide3/1
  Constant2/1 -> Divide3/2
  Divide3/1 -> Length Conversion/1
  Sum1/1 -> "Altitude, m"/1
  Sum2/1 -> Divide/1
  Length Conversion/1 -> Sum1/1

== system ReplayFlight_ALL_PARMS_v6/Sensor Data/Sensor Suite/Low Pass Filtering,Temperature Compensation and Calibration/Baro Altimeter/Enabled Subsystem ==
  In1 : Inport  OutDataType=sfix(16)  OutScaling=2^0
  Enable : EnablePort
  Out1 : Outport  OutDataType=sfix(16)  OutScaling=2^0  InitialOutput=baseHeight
  wires:
  In1/1 -> Out1/1

== system ReplayFlight_ALL_PARMS_v6/Sensor Data/Sensor Suite/Low Pass Filtering,Temperature Compensation and Calibration/Baro Altimeter/Initial Baro Bias ==
  Baro (Pa) : Inport  OutDataType=sfix(16)  OutScaling=2^0
  Enable : EnablePort
  Data Type Conversion : DataTypeConversion  OutDataTypeMode=double  OutDataType=sfix(16)  OutScaling=2^0  OutDataTypeStr=double
  Data Type Conversion1 : DataTypeConversion  OutDataTypeMode=single  OutDataType=sfix(16)  OutScaling=2^0  OutDataTypeStr=single
  Low Pass8 : Subsystem  mask(DiscretizedZeroPole){Zeros=[], Poles=[-3], Gain=3, AbsTol=auto, SampleTime=.01, method=tustin, Wc=1}
      mask prompts: Zeros "Zeros (enter in s-main:)"; Poles "Poles (enter in s-domain:)"; Gain "Gain (enter in s-domain:)"; AbsTol "Absolute tolerance:"; SampleTime "Sample time:"; Wc "Critical Frequency (Hz):"
      mask help: Continuous mask uses c2d to transform parameters onto the Discrete Zero-Pole block inside.
      mask init: same as ReplayFlight_ALL_PARMS_v6/Position and Attitude Filter/Attitude Complimentary Filter COG/3D Filter/Filter1
      mask StyleString: edit,edit,edit,edit,edit,popup(zoh|foh|tustin|prewarp|matched),edit
      mask CallbackString: |||||hidecrit|
      mask Display:
      | droots(zeross,poless,gainss)
      | text( 0.5, 1.0, method, 'verticalAlignment','top')
  Mux : Mux  Inputs=2
  Scope : Scope
      settings: SaveName=ScopeData8
  "[80k - 120k]" : Saturate  UpperLimit=120000  LowerLimit=80000
  Baro (Gnd) : Outport  OutDataType=sfix(16)  OutScaling=2^0
  wires:
  "[80k - 120k]"/1 -> Mux/1, Baro (Gnd)/1
  Mux/1 -> Scope/1
  Data Type Conversion1/1 -> "[80k - 120k]"/1, Mux/2
  Data Type Conversion/1 -> Low Pass8/1(In1)
  Low Pass8/1(Out1) -> Data Type Conversion1/1
  Baro (Pa)/1 -> Data Type Conversion/1

== system ReplayFlight_ALL_PARMS_v6/Sensor Data/Sensor Suite/Low Pass Filtering,Temperature Compensation and Calibration/Baro Altimeter/Zero Out Height ==
  Base Height : Inport  OutDataType=sfix(16)  OutScaling=2^0
  Computed Height : Inport  Port=2  OutDataType=sfix(16)  OutScaling=2^0
  Enable : EnablePort
  Integer Delay : simulink/Discrete/Integer Delay  vinit=0  samptime=.01  NumDelays=1
  Sum : Sum  Inputs=|+-  OutDataTypeMode=single  OutDataType=sfix(16)  OutScaling=2^0  OutDataTypeStr=single
  Height Offset : Outport  OutDataType=sfix(16)  OutScaling=2^0
  wires:
  Base Height/1 -> Sum/1
  Integer Delay/1 -> Sum/2
  Sum/1 -> Height Offset/1
  Computed Height/1 -> Integer Delay/1

== system ReplayFlight_ALL_PARMS_v6/Sensor Data/Sensor Suite/Low Pass Filtering,Temperature Compensation and Calibration/Temp Compensate Accel X1/Hi Temp Compensation2 ==
  Raw : Inport  OutDataType=sfix(16)  OutScaling=2^0
  Temp Raw : Inport  Port=2  OutDataType=sfix(16)  OutScaling=2^0
  Enable : EnablePort
  Divide1 : Product  OutDataTypeMode=single  OutDataType=sfix(16)  OutScaling=2^-10  OutDataTypeStr=single
  Mean Temperature for Calibration : Constant  Value=tempMean  OutDataTypeMode=single  OutDataType=sfix(16)  OutScaling=2^0  OutDataTypeStr=single
  Sum1 : Sum  Inputs=|+-  OutDataTypeMode=single  OutDataType=sfix(16)  OutScaling=2^0  OutDataTypeStr=single
  Sum2 : Sum  Inputs=|+-  OutDataTypeMode=single  OutDataType=sfix(16)  OutScaling=2^0  OutDataTypeStr=single
  gains : Constant  Value=alpha  OutDataTypeMode=single  OutDataType=sfix(16)  OutScaling=2^0  OutDataTypeStr=single
  Comp : Outport  OutDataType=sfix(16)  OutScaling=2^0
  wires:
  Sum2/1 -> Comp/1
  Divide1/1 -> Sum2/2
  gains/1 -> Divide1/1
  Sum1/1 -> Divide1/2
  Temp Raw/1 -> Sum1/1
  Raw/1 -> Sum2/1
  Mean Temperature for Calibration/1 -> Sum1/2

== system ReplayFlight_ALL_PARMS_v6/Sensor Data/Sensor Suite/Low Pass Filtering,Temperature Compensation and Calibration/Temp Compensate Accel X1/Lo Temp Compensation ==
  Raw : Inport  OutDataType=sfix(16)  OutScaling=2^0
  Temp Raw : Inport  Port=2  OutDataType=sfix(16)  OutScaling=2^0
  Enable : EnablePort
  Add : Sum  OutDataTypeMode=single  OutDataType=sfix(16)  OutScaling=2^-10  OutDataTypeStr=single
  Constant : Constant  Value=pitAdjust  OutDataTypeMode=single  OutDataType=sfix(16)  OutScaling=2^0  OutDataTypeStr=single
  Divide1 : Product  OutDataTypeMode=single  OutDataType=sfix(16)  OutScaling=2^-10  OutDataTypeStr=single
  Mean Temperature for Calibration : Constant  Value=tempMean  OutDataTypeMode=single  OutDataType=sfix(16)  OutScaling=2^0  OutDataTypeStr=single
  Sum1 : Sum  Inputs=|+-  OutDataTypeMode=single  OutDataType=sfix(16)  OutScaling=2^0  OutDataTypeStr=single
  Sum2 : Sum  Inputs=|+-  OutDataTypeMode=single  OutDataType=sfix(16)  OutScaling=2^0  OutDataTypeStr=single
  gains : Constant  Value=alpha  OutDataTypeMode=single  OutDataType=sfix(16)  OutScaling=2^0  OutDataTypeStr=single
  Comp : Outport  OutDataType=sfix(16)  OutScaling=2^0
  wires:
  Mean Temperature for Calibration/1 -> Sum1/2
  Raw/1 -> Sum2/1
  Temp Raw/1 -> Sum1/1
  Sum1/1 -> Divide1/2
  gains/1 -> Divide1/1
  Divide1/1 -> Sum2/2
  Sum2/1 -> Add/1
  Constant/1 -> Add/2
  Add/1 -> Comp/1

== system ReplayFlight_ALL_PARMS_v6/Sensor Data/Sensor Suite/Low Pass Filtering,Temperature Compensation and Calibration/Temp Compensate Baro/Hi Temp Compensation ==
  Raw : Inport  OutDataType=sfix(16)  OutScaling=2^0
  Temp Raw : Inport  Port=2  OutDataType=sfix(16)  OutScaling=2^0
  Enable : EnablePort
  Add : Sum  OutDataTypeMode=single  OutDataType=sfix(16)  OutScaling=2^-10  OutDataTypeStr=single
  Constant : Constant  Value=barAdjust  OutDataTypeMode=single  OutDataType=sfix(16)  OutScaling=2^0  OutDataTypeStr=single
  Divide1 : Product  OutDataTypeMode=single  OutDataType=sfix(16)  OutScaling=2^-10  OutDataTypeStr=single
  Mean Temperature for Calibration : Constant  Value=tempMean  OutDataTypeMode=single  OutDataType=sfix(16)  OutScaling=2^0  OutDataTypeStr=single
  Sum1 : Sum  Inputs=|+-  OutDataTypeMode=single  OutDataType=sfix(16)  OutScaling=2^0  OutDataTypeStr=single
  Sum2 : Sum  Inputs=|+-  OutDataTypeMode=single  OutDataType=sfix(16)  OutScaling=2^0  OutDataTypeStr=single
  gains : Constant  Value=alpha  OutDataTypeMode=single  OutDataType=sfix(16)  OutScaling=2^0  OutDataTypeStr=single
  Comp : Outport  OutDataType=sfix(16)  OutScaling=2^0
  wires:
  Mean Temperature for Calibration/1 -> Sum1/2
  Raw/1 -> Sum2/1
  Temp Raw/1 -> Sum1/1
  Sum1/1 -> Divide1/2
  gains/1 -> Divide1/1
  Divide1/1 -> Sum2/2
  Constant/1 -> Add/1
  Add/1 -> Comp/1
  Sum2/1 -> Add/2

== system ReplayFlight_ALL_PARMS_v6/Sensor Data/Sensor Suite/Low Pass Filtering,Temperature Compensation and Calibration/Temp Compensate Baro/Lo Temp Compensation ==
  Raw : Inport  OutDataType=sfix(16)  OutScaling=2^0
  Temp Raw : Inport  Port=2  OutDataType=sfix(16)  OutScaling=2^0
  Enable : EnablePort
  Divide1 : Product  OutDataTypeMode=single  OutDataType=sfix(16)  OutScaling=2^-10  OutDataTypeStr=single
  Mean Temperature for Calibration : Constant  Value=tempMean  OutDataTypeMode=single  OutDataType=sfix(16)  OutScaling=2^0  OutDataTypeStr=single
  Sum1 : Sum  Inputs=|+-  OutDataTypeMode=single  OutDataType=sfix(16)  OutScaling=2^0  OutDataTypeStr=single
  Sum2 : Sum  Inputs=|+-  OutDataTypeMode=single  OutDataType=sfix(16)  OutScaling=2^0  OutDataTypeStr=single
  gains : Constant  Value=alpha  OutDataTypeMode=single  OutDataType=sfix(16)  OutScaling=2^0  OutDataTypeStr=single
  Comp : Outport  OutDataType=sfix(16)  OutScaling=2^0
  wires:
  Sum2/1 -> Comp/1
  Divide1/1 -> Sum2/2
  gains/1 -> Divide1/1
  Sum1/1 -> Divide1/2
  Temp Raw/1 -> Sum1/1
  Raw/1 -> Sum2/1
  Mean Temperature for Calibration/1 -> Sum1/2

== system ReplayFlight_ALL_PARMS_v6/Sensor Data/Sensor Suite/Low Pass Filtering,Temperature Compensation and Calibration/ValidateMags/Hold if Outlier ==
  In1 : Inport  OutDataType=sfix(16)  OutScaling=2^0
  Enable : EnablePort
  Out1 : Outport  OutDataType=sfix(16)  OutScaling=2^0  OutputWhenDisabled=reset  InitialOutput=[0 0 0]
  wires:
  In1/1 -> Out1/1

== system ReplayFlight_ALL_PARMS_v6/Sensor Data/Sensor Suite/Low Pass Filtering,Temperature Compensation and Calibration/ValidateMags/Monitor Norm ==
  Mags : Inport  OutDataType=sfix(16)  OutScaling=2^0
  0.7 < Norm < 1.5 : Subsystem
  Norm : Subsystem  AncestorBlock=SLUGS_Library/Navigation/Norm
  Enable : Outport  OutDataType=sfix(16)  OutScaling=2^0
  wires:
  Mags/1 -> Norm/1(Vector)
  0.7 < Norm < 1.5/1(flag) -> Enable/1
  Norm/1(Norm) -> 0.7 < Norm < 1.5/1(norm)

== system ReplayFlight_ALL_PARMS_v6/Position and Attitude Filter/Attitude Complimentary Filter COG/DoParmTests/AngleAxis_Test/CreateAngleAxisDot/Skew symmetric matrix ==
  axis_in : Inport  PortDimensions=3  SampleTime=SampleT  DataType=single  OutDataType=fixdt(1, 16)  OutScaling=2^0  OutDataTypeStr=single
  Constant : Constant  Value=0  OutDataTypeMode=single  OutDataType=fixdt(1, 16)  OutScaling=2^0  OutDataTypeStr=single
  Constant1 : Constant  Value=0  OutDataTypeMode=single  OutDataType=fixdt(1, 16)  OutScaling=2^0  OutDataTypeStr=single
  Constant2 : Constant  Value=0  OutDataTypeMode=single  OutDataType=fixdt(1, 16)  OutScaling=2^0  OutDataTypeStr=single
  Demux : Demux  Outputs=3
  Gain : Gain  Gain=-1  ParameterDataType=fixdt(1, 16)  ParameterScaling=2^0  OutDataTypeMode=single  OutDataType=fixdt(1, 16)  OutScaling=2^0  OutDataTypeStr=single
  Gain1 : Gain  Gain=-1  ParameterDataType=fixdt(1, 16)  ParameterScaling=2^0  OutDataTypeMode=single  OutDataType=fixdt(1, 16)  OutScaling=2^0  OutDataTypeStr=single
  Gain2 : Gain  Gain=-1  ParameterDataType=fixdt(1, 16)  ParameterScaling=2^0  OutDataTypeMode=single  OutDataType=fixdt(1, 16)  OutScaling=2^0  OutDataTypeStr=single
  Mux{,1..3} (4 alike) : Mux  Inputs=3
  Reshape : Reshape  OutputDimensionality=Customize  OutputDimensions=[3,3]
  axis_x : Outport  PortDimensions=[3,3]  SampleTime=SampleT  DataType=single  OutDataType=fixdt(1, 16)  OutScaling=2^0  OutDataTypeStr=single
  wires:
  axis_in/1 -> Demux/1
  Reshape/1 -> axis_x/1
  Constant/1 -> Mux/1
  Demux/3 -> Mux/2, Gain1/1
  Demux/2 -> Gain/1, Mux2/1
  Constant1/1 -> Mux1/2
  Demux/1 -> Mux1/3, Gain2/1
  Constant2/1 -> Mux2/3
  Mux/1 -> Mux3/1
  Mux1/1 -> Mux3/2
  Mux2/1 -> Mux3/3
  Mux3/1 -> Reshape/1
  Gain/1 -> Mux/3
  Gain1/1 -> Mux1/1
  Gain2/1 -> Mux2/2

== system ReplayFlight_ALL_PARMS_v6/Position and Attitude Filter/Attitude Complimentary Filter COG/DoParmTests/DCM Tests/Murray_Mexp/Skew symmetric matrix ==
  omega_in : Inport  PortDimensions=3  SampleTime=SampleT  OutDataType=fixdt(1, 16)  OutScaling=2^0
  Constant : Constant  Value=0  OutDataTypeMode=single  OutDataType=fixdt(1, 16)  OutScaling=2^0  OutDataTypeStr=single
  Constant1 : Constant  Value=0  OutDataTypeMode=single  OutDataType=fixdt(1, 16)  OutScaling=2^0  OutDataTypeStr=single
  Constant2 : Constant  Value=0  OutDataTypeMode=single  OutDataType=fixdt(1, 16)  OutScaling=2^0  OutDataTypeStr=single
  Demux : Demux  Outputs=3
  Gain : Gain  Gain=-1  ParameterDataType=fixdt(1, 16)  ParameterScaling=2^0  OutDataType=fixdt(1, 16)  OutScaling=2^0
  Gain1 : Gain  Gain=-1  ParameterDataType=fixdt(1, 16)  ParameterScaling=2^0  OutDataType=fixdt(1, 16)  OutScaling=2^0
  Gain2 : Gain  Gain=-1  ParameterDataType=fixdt(1, 16)  ParameterScaling=2^0  OutDataType=fixdt(1, 16)  OutScaling=2^0
  Mux{,1..3} (4 alike) : Mux  Inputs=3
  Reshape : Reshape  OutputDimensionality=Customize  OutputDimensions=[3,3]
  omega_x : Outport  PortDimensions=[3,3]  SampleTime=SampleT  OutDataType=fixdt(1, 16)  OutScaling=2^0
  wires:
  omega_in/1 -> Demux/1
  Reshape/1 -> omega_x/1
  Constant/1 -> Mux/1
  Demux/3 -> Mux/2, Gain1/1
  Demux/2 -> Gain/1, Mux2/1
  Constant1/1 -> Mux1/2
  Demux/1 -> Mux1/3, Gain2/1
  Constant2/1 -> Mux2/3
  Mux/1 -> Mux3/1
  Mux1/1 -> Mux3/2
  Mux2/1 -> Mux3/3
  Mux3/1 -> Reshape/1
  Gain/1 -> Mux/3
  Gain1/1 -> Mux1/1
  Gain2/1 -> Mux2/2
